simulink model "bsp_nxt_touch"  (R2019a)
settings: Solver=FixedStepAuto  StartTime=0.0  StopTime=20  FixedStep=0.1  RelTol=1e-3  EnableMultiTasking=on
libraries: BrickPiSimSubLib_getsensor x1, BrickPiSimSubLib_initreset x1
settings Model: Creator=uk008555  LastModifiedBy=uk008555
settings SolverCC: PositivePriorityOrder=on
settings OptimizationCC: EnhancedBackFolding=on  PassReuseOutputArgsAs=Individual arguments  MaxStackSize=64  OptimizeBlockOrder=speed  DifferentSizesBufferReuse=on  OptimizationCustomize=off
settings DebuggingCC: ParameterTunabilityLossMsg=error
settings HardwareCC: ProdBitPerPointer=32  ProdBitPerSizeT=32  ProdBitPerPtrDiffT=32  ProdLargestAtomicInteger=Long  ProdLargestAtomicFloat=Double  ProdWordSize=32  ProdLongLongMode=on  ProdHWDeviceType=ARM Compatible->ARM Cortex
settings SFSimCC: MATLABDynamicMemAlloc=off
settings RTWCC: SystemTargetFile=ert.tlc  HardwareBoard=Raspberry Pi  TLCOptions="-aInlineSetEventsForThisBaseRateFcn=TLC_FALSE -aSuppressMultiTaskScheduler=TLC_FALSE  -aRateBasedStepFcn=0"  TemplateMakefile=ert_default_tmf  GenerateReport=on  Toolchain=GNU GCC Raspberry Pi  BuildConfiguration=Faster Runs  IncludeHyperlinkInReport=on  LaunchReport=on  GenerateTraceInfo=on  GenerateTraceReport=on  GenerateTraceReportSl=on  GenerateTraceReportSf=on  GenerateTraceReportEml=on
settings CodeAppCC: ForceParamTrailComments=on  IgnoreCustomStorageClasses=off  OperatorAnnotations=on  SimulinkDataObjDesc=on  SFDataObjDesc=on  InsertBlockDesc=on
settings ERTTargetCC: SupportVariableSizeSignals=on

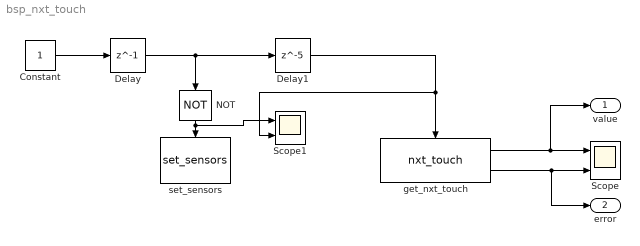
== system bsp_nxt_touch ==
  Constant : Constant
  Delay : Delay  DelayLength=1
  Delay1 : Delay  DelayLength=5
  NOT : Logic  Operator=NOT  IconShape=distinctive  AllPortsSameDT=off  OutDataTypeStr=boolean
  Scope : Scope  NumInputPorts=2
  Scope1 : Scope  NumInputPorts=2
  get_nxt_touch : BrickPiSimSubLib_getsensor/nxt_touch  Add_Val=1  Port_Val=2
      settings: SourceProductName=Simulink Support Package for BrickPi
  set_sensors : BrickPiSimSubLib_initreset/set_sensors  Add_Val=1  Type_Val=Touch NXT  Port1_Val=off  Port2_Val=on  Port3_Val=off  Port4_Val=off
      settings: SourceProductName=Simulink Support Package for BrickPi
  value : Outport
  error : Outport  Port=2
  wires:
  get_nxt_touch/1 -> value/1, Scope/1
  get_nxt_touch/2 -> Scope/2, error/1
  Constant/1 -> Delay/1
  Delay/1 -> NOT/1, Delay1/1
  Delay1/1 -> get_nxt_touch/Enable, Scope1/2
  NOT/1 -> Scope1/1, set_sensors/Enable
